simulink model "test_npn_gen"  (Simulink 7.7)
settings: Solver=FixedStepDiscrete  StartTime=0.0  StopTime=10000.0  FixedStep=1  RelTol=1e-3
libraries: SimpleModeling x3
settings Model: Creator=medcps  LastModifiedBy=iris
settings DataIOCC: SaveFormat=StructureWithTime  SignalLogging=off
settings OptimizationCC: BlockReduction=off  ConditionallyExecuteInputs=off  InlineParams=on
settings DebuggingCC: AlgebraicLoopMsg=error  FcnCallInpInsideContextMsg=Enable All
settings HardwareCC: ProdHWDeviceType=ASIC/FPGA->ASIC/FPGA

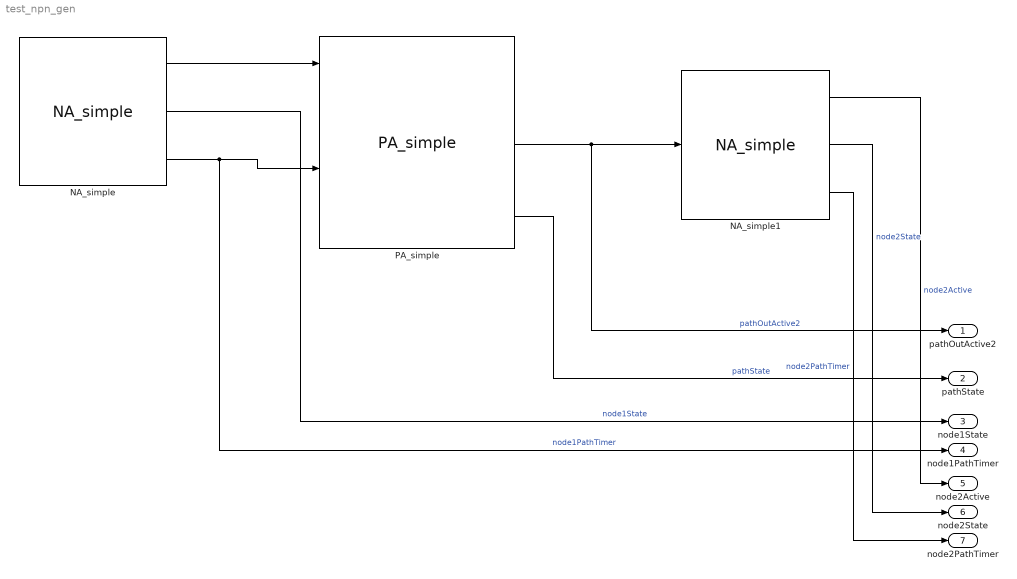
== system test_npn_gen ==
  NA_simple : SimpleModeling/NA_simple  SystemSampleTime=-1  TERP_defs=0  TRRP_def=100  Trest_def=800  TERP_s=320  TRRP_s=100  Trest_s=800  Terp_min=150  Terp_max=300
  NA_simple1 : SimpleModeling/NA_simple  SystemSampleTime=-1  TERP_defs=0  TRRP_def=120  Trest_def=9999  TERP_s=320  TRRP_s=100  Trest_s=800  Terp_min=150  Terp_max=300
  PA_simple : SimpleModeling/PA_simple  SystemSampleTime=-1  min_path_par=10  bck_param=36  forw_param=36
  pathOutActive2 : Outport
  pathState : Outport  Port=2
  node1State : Outport  Port=3
  node1PathTimer : Outport  Port=4
  node2Active : Outport  Port=5
  node2State : Outport  Port=6
  node2PathTimer : Outport  Port=7
  wires:
  NA_simple/1 -> PA_simple/1
  NA_simple/3 -> PA_simple/3, node1PathTimer/1  "node1PathTimer"
  PA_simple/2 -> NA_simple1/1, pathOutActive2/1  "pathOutActive2"
  PA_simple/3 -> pathState/1  "pathState"
  NA_simple/2 -> node1State/1  "node1State"
  NA_simple1/1 -> node2Active/1  "node2Active"
  NA_simple1/2 -> node2State/1  "node2State"
  NA_simple1/3 -> node2PathTimer/1  "node2PathTimer"
